simulink model "ng_pv_dynamic_dbus_p_3_ss_dbus"  (Simulink 8.8)
settings: Solver=ode4  StartTime=0.0  StopTime=inf  FixedStep=0.000125  RelTol=1e-3  EnableMultiTasking=on
PreLoadFcn:
  | Ts=125e-6;Core_Num = 0; np=1; nq=1; Vmin=.9;
PostLoadFcn:
  | Ts=125e-6;Core_Num = 0; np=1; nq=1; Vmin=.9;
InitFcn:
  | Ts=125e-6;Core_Num = 0; np=1; nq=1; Vmin=.9;
libraries: opal_lib x5, artemis x1, rtio_generic_ethernet x1, powerlib x1
settings Model: ARTEMISmethode_block_infos=$$__separator__$$ng_pv_dynamic_dbus_p_3_ss_dbus/ARTEMIS Guide1$$__separator__$$  Creator=DETLDAQ  LastModifiedBy=DETLDAQ
settings OptimizationCC: BlockReduction=off  BooleanDataType=off  OptimizeBlockIOStorage=off  BufferReuse=off  GlobalBufferReuse=off  ExpressionFolding=off  LocalBlockOutputs=off
settings DebuggingCC: SaveWithParameterizedLinksMsg=none  SignalResolutionControl=TryResolveAllWithWarning  MultiTaskDSMMsg=warning  MultiTaskCondExecSysMsg=none  FcnCallInpInsideContextMsg=error
settings HardwareCC: TargetBitPerPointer=64  TargetBitPerSizeT=64  TargetBitPerPtrDiffT=64  TargetLongLongMode=on  TargetIntDivRoundTo=Zero  TargetEndianess=LittleEndian  TargetWordSize=64  TargetHWDeviceType=MATLAB Host  ProdEqTarget=off
settings RTWCC: GenCodeOnly=on
settings GRTTargetCC: CombineOutputUpdateFcns=on  GRTInterface=off

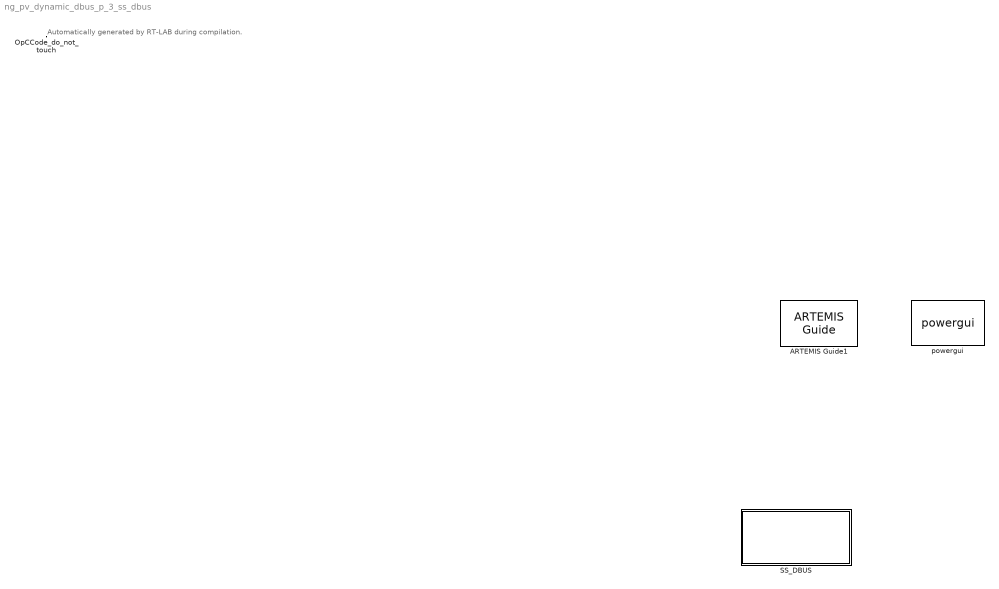
== system ng_pv_dynamic_dbus_p_3_ss_dbus ==
  note: Automatically generated by RT-LAB during compilation.
  ARTEMIS Guide1 : artemis/ARTEMIS/ARTEMIS Guide  Tag=FTSSmethode_opal_4hx0r99  Description=5.0_z1  lock=on  Ts=Ts  opt=art5  dyna=off  nb_perm=4  RT_fullcomp=off  ssn=on  ssn_itvc=off  ssn_ivic=off  ssn_ext=off  ssn_solver=Backward Euler  ssn_impulse=off  ssn_quasimpulse=off  ssn_impulse_loop=5  paraExtinctionThy=off  Thy_Impulse=off  dtc=Off  dtc_opt=normal  ao=on  simtype=off  ct_mac=off  lin_mov=off  lsp=[0.001 2]  spike_skip=Disabled  dtc_extra=1  dtc_sws=normal  dtc_pied=0.5  SPSRulesBlock=SPSRules  tre=off  ctmm=off  LF=on  dpl_type=ARTEMiS DPL  rlc_type=off  custom_type=off  para=on  ssn_ImpulseLoopBlockedStateUpdate=5  ssn_mov_iter_number=5  ssn_switch_iter_number=5  ssn_nib_type_verify=on  ssn_use_lu=on  ssn_use_ldlt=off
  OpCCode_do_not_touch : opal_lib/Communication/OpCCode  SystemSampleTime=-1
  SS_DBUS : Subsystem
  powergui : powerlib/powergui  SimulationMode=Discrete  SolverType=Backward Euler  SampleTime=0.000125  frequency=60  SPID=off  DisableSnubberDevices=off  DisableRonSwitches=off  DisableVfSwitches=off  SwTol=0  DisplayEquations=off  Interpol=off  ExternalGateDelay=off  methode=off  Ts=100  FunctionMessages=off  echomessages=off  HookPort=off  EnableUseOfTLC=off  x0status=blocks  frequencyindice=0  Pbase=100e6  ErrMax=1e-4  Iterations=50  UnitsV=kV  UnitsW=MW  buscounter=0  RestoreLinks=warning  ResistiveCurrentMeasurement=off  Frange=[0:2:500]  Ylog=off  Xlog=on  ShowGrid=off  save=off  variable=ZData  structure=0  ZoomFFT=off  StartTime=0.0  cycles=1  DisplayStyle=1  fundamental=60  FreqAxis=off  MaxFrequency=1000  frequencyindicesteady=1  RmsSteady=1  display=off

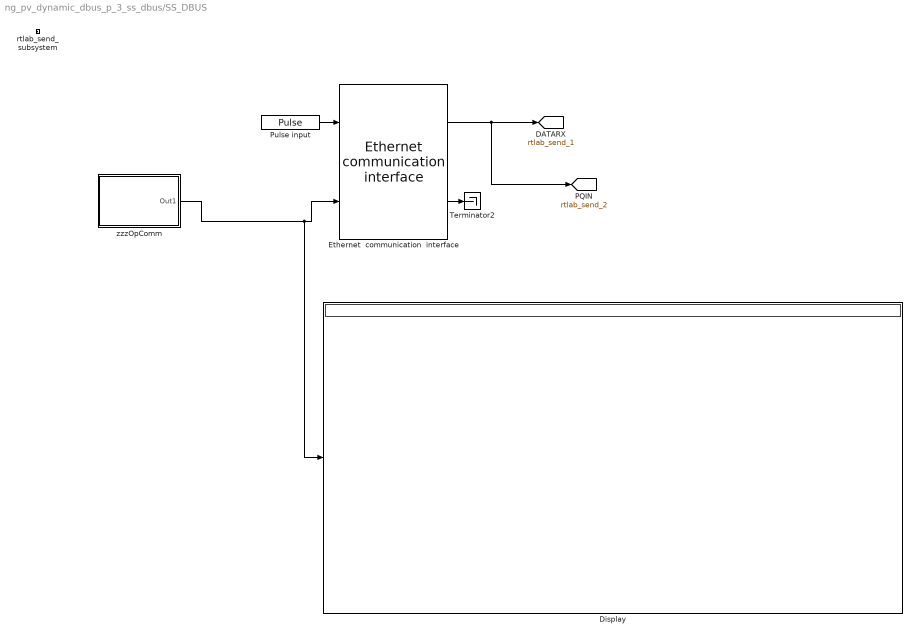
== system ng_pv_dynamic_dbus_p_3_ss_dbus/SS_DBUS ==
  Display : Display
  Ethernet  communication  interface : rtio_generic_ethernet/Ethernet communication interface  ctrl_id=1  nbr_to_remote_endpoint=64  type_to_remote_endpoint=FLOAT  offset_to_remote_endpoint=0  swap_tx=on  nbr_from_remote_endpoint=62  type_from_remote_endpoint=FLOAT  offset_from_remote_endpoint=0  swap_rx=on  exe_name='AsyncEthernet'  nic_name='eth0'  protocol=TCP  tcp_mode=Client  port=6340  remote_ip='10.1.2.2'
  Pulse input : DiscretePulseGenerator  Period=round(1/Ts)  SampleTime=Ts
  Terminator2 : Terminator
  rtlab_send_subsystem : Subsystem  Priority=-100
      mask Display: text(0,0,'');
  zzzOpComm : Subsystem
      mask init:
      | opmaskdisplay('maskdisplay_block',gcb,'disp(''OpComm'')');
      mask Display:
      | patch([0 0.5 0.7 0],[1 1 0 0],[0.7 0.75 0.9]);
      | patch([1 0.53 0.73 1],[1 1 0 0],[1 0.8 0.7]);
      | plot([0 0 1 1 0],[0 1 1 0 0]);
      | disp('OpComm')
  tag scope: rtlab_send_1=global, rtlab_send_2=global
  wires:
  Ethernet  communication  interface/2 -> Terminator2/1
  Pulse input/1 -> Ethernet  communication  interface/1
  Ethernet  communication  interface/1 -> [rtlab_send_2], [rtlab_send_1]
  zzzOpComm/1(Out1) -> Display/1, Ethernet  communication  interface/2

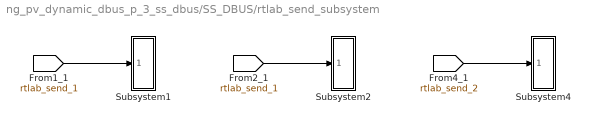
== system ng_pv_dynamic_dbus_p_3_ss_dbus/SS_DBUS/rtlab_send_subsystem ==
  Subsystem1 : Subsystem
  Subsystem2 : Subsystem  Priority=-200000  TreatAsAtomicUnit=on
  Subsystem4 : Subsystem  Priority=-200000  TreatAsAtomicUnit=on
  wires:
  [rtlab_send_1] -> Subsystem1/1(In1)
  [rtlab_send_1] -> Subsystem2/1(In1)
  [rtlab_send_2] -> Subsystem4/1(In1)

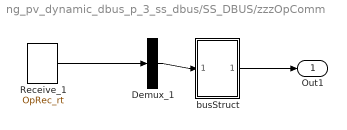
== system ng_pv_dynamic_dbus_p_3_ss_dbus/SS_DBUS/zzzOpComm ==
  Demux_1 : Demux  Outputs=[64]
  Receive_1 : opal_lib/Communication/OpRec_rt  src=1  Data_width=64  st=0.000125
  busStruct : Subsystem
  Out1 : Outport
  wires:
  Demux_1/1 -> busStruct/1(In1)
  busStruct/1(Out1) -> Out1/1
  Receive_1/1 -> Demux_1/1

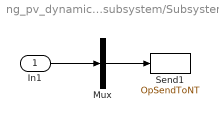
== system ng_pv_dynamic_dbus_p_3_ss_dbus/SS_DBUS/rtlab_send_subsystem/Subsystem1 ==
  In1 : Inport
  Mux : Mux  Inputs=1
  Send1 : opal_lib/Communication/OpSendToNT  Acqu_group=1
  wires:
  Mux/1 -> Send1/1
  In1/1 -> Mux/1

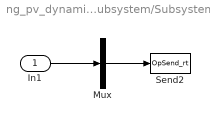
== system ng_pv_dynamic_dbus_p_3_ss_dbus/SS_DBUS/rtlab_send_subsystem/Subsystem2 ==
  In1 : Inport
  Mux : Mux  Inputs=1
  Send2 : opal_lib/Communication/OpSend_rt  dest=1  priority2=0  st=0.000125
  wires:
  Mux/1 -> Send2/1
  In1/1 -> Mux/1

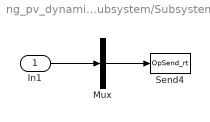
== system ng_pv_dynamic_dbus_p_3_ss_dbus/SS_DBUS/rtlab_send_subsystem/Subsystem4 ==
  In1 : Inport
  Mux : Mux  Inputs=1
  Send4 : opal_lib/Communication/OpSend_rt  dest=4  priority2=0  st=0.000125
  wires:
  Mux/1 -> Send4/1
  In1/1 -> Mux/1

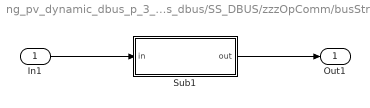
== system ng_pv_dynamic_dbus_p_3_ss_dbus/SS_DBUS/zzzOpComm/busStruct ==
  In1 : Inport
  Sub1 : Subsystem
  Out1 : Outport
  wires:
  Sub1/1(out) -> Out1/1
  In1/1 -> Sub1/1(in)

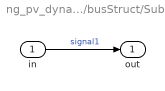
== system ng_pv_dynamic_dbus_p_3_ss_dbus/SS_DBUS/zzzOpComm/busStruct/Sub1 ==
  in : Inport
  out : Outport
  wires:
  in/1 -> out/1  "signal1"
